simulink model "Appl_HeatAdj_CtrlModel"  (R2018b)
settings: configuration reference "CodeConfig_10_ms" (kept outside this file)
undefined symbols (not defined in the file): CAL_LEVEL3_TIMEOUT, CAL_SW_20min_TIMEOUT, D_1stLevel_36, D_2ndLevel_39, D_3rdLevel_45, D_3rdLevel_48, D_DRVHEAT_PID_D, D_DRVHEAT_PID_I, D_DRVHEAT_PID_P, D_HEAT_HEAT_DEF, D_SwsLevel_Temp, FALSE, TRUE
libraries: DareLib x111, simulink x1
(part 4 of 6)

== stateflow chart Appl_HeatAdj_CtrlModel/LogicCtrl/LocalAdjustCtrl/LimitDeal/LevelLimitFunction/LevelLimit ==
  state Default
    en:
    Level = enHeatLvlSts.EN_HEAT_LVL_OFF;
  state Run
    en:
    Level = OriginalLevel;
    CANStopReason = enHeatStopReason.EN_HEAT_STOP_R_NONE;
    du:
    Level = OriginalLevel;
  state ForbidStatus
    en:
    Level = enHeatLvlSts.EN_HEAT_LVL_OFF;
    CANStopReason = StopReason;
    //暂时屏蔽，查看是否需要一直保存禁能原因
    ex:
    StopReason = enHeatStopReason.EN_HEAT_STOP_R_NONE;
    (default) -> (junction 34)
    ForbidStatus -> (junction 34) [order 1]
    (junction 34) -> (junction 37) [order 1] : /*存在故障*/
        | [TRUE == Error]
    (junction 34) -> (junction 41) [order 2]
    (junction 37) -> (junction 39) : {StopReason = enHeatStopReason.EN_HEAT_STOP_R_FAULT;}
    (junction 39) -> (junction 41)
    (junction 41) -> (junction 44)
    (junction 44) -> (junction 46) [order 1] : /*互斥命令有效*/
        | [TRUE == OppositeCmd]
    (junction 44) -> (junction 50) [order 2]
    (junction 46) -> (junction 48) : {StopReason = enHeatStopReason.EN_HEAT_STOP_R_CMD;}
    (junction 48) -> (junction 50)
    (junction 50) -> (junction 62)
    (junction 62) -> (junction 60) [order 1] : /*恢复出厂*/
        | [TRUE == Heat_RecoverDefaultFlag]
    (junction 62) -> (junction 55) [order 2]
    (junction 60) -> (junction 58) : {StopReason = enHeatStopReason.EN_HEAT_STOP_R_FACTORY;}
    (junction 58) -> (junction 55)
    (junction 55) -> (junction 71)
    (junction 71) -> (junction 69) [order 1] : /*BM400掉线禁能*/
        | [TRUE == Heat_CanMessageLostFlag && enProjectType.EN_PROJECT_BM400 == CarType]
    (junction 71) -> (junction 67) [order 2]
    (junction 69) -> (junction 64) : {StopReason = enHeatStopReason.EN_HEAT_STOP_R_LOSS;}
    (junction 64) -> (junction 67)
    (junction 67) -> (junction 73)
  (default) -> Default
  ForbidStatus -> Default [order 1] : /*无用户请求，可准备下一轮禁能原因检测*/
      | [enHeatLvlSts.EN_HEAT_LVL_OFF == OriginalLevel]
  Default -> ForbidStatus : /*请求工作*/
      | [enHeatLvlSts.EN_HEAT_LVL_OFF != OriginalLevel]
  Run -> ForbidStatus [order 1] : /*存在故障*/
      | [TRUE == Error]
      | /StopReason = enHeatStopReason.EN_HEAT_STOP_R_FAULT;
  Run -> ForbidStatus [order 2] : /*互斥命令有效*/
      | [TRUE == OppositeCmd]
      | /StopReason = enHeatStopReason.EN_HEAT_STOP_R_CMD;
  Run -> ForbidStatus [order 3] : /*恢复出厂*/
      | [TRUE == Heat_RecoverDefaultFlag]
      | /StopReason = enHeatStopReason.EN_HEAT_STOP_R_FACTORY;
  Run -> ForbidStatus [order 4] : /*BM400掉线禁能*/
      | [TRUE == Heat_CanMessageLostFlag && enProjectType.EN_PROJECT_BM400 == CarType]
      | /StopReason = enHeatStopReason.EN_HEAT_STOP_R_LOSS;
  ForbidStatus -> Run [order 2] : /*无故障
      | && 互斥命令无效
      | && 无恢复出厂命令
      | && （BM400控制报文在线 || 非BM400车型）*/
      | [TRUE != Error ...
      | && TRUE != OppositeCmd ...
      | && TRUE != Heat_RecoverDefaultFlag ...
      | && ((FALSE == Heat_CanMessageLostFlag && enProjectType.EN_PROJECT_BM400 == CarType) ...
      | || (enProjectType.EN_PROJECT_BM400 != CarType))]
      | /StopReason = enHeatStopReason.EN_HEAT_STOP_R_NONE
  data: Level output Enum: enHeatLvlSts; StopReason output Enum: enHeatStopReason; OriginalLevel input Enum: enHeatLvlSts; Error input uint8; CarType input Enum: enProjectType; TRUE parameter; OppositeCmd input uint8; Heat_CanMessageLostFlag input uint8; Heat_RecoverDefaultFlag input uint8; FALSE parameter; CANStopReason output Enum: enHeatStopReason

== stateflow chart Appl_HeatAdj_CtrlModel/LogicCtrl/LocalAdjustCtrl/LimitDeal/TimeoutFunction1/Timeout ==
  state Ts = D_HAL_GET_CUR_MS_TS [function]
  state OutTs = TimeDiffTs(lastTs,Ts) [function]
  state TimeCountStatus
    state TimeoutSts
      en:
      Level = enHeatLvlSts.EN_HEAT_LVL_OFF;
      du:
      Level = enHeatLvlSts.EN_HEAT_LVL_OFF;
      ex:
      Timer = 0;
    state Init
      en:
      Level = InLevel;
      Timer = D_HAL_GET_CUR_MS_TS();
      du:
      Level = InLevel;
      ex:
      Timer = D_HAL_GET_CUR_MS_TS();
    (default) -> Init
    Init -> TimeoutSts [order 1] : [TimeDiffTs(Timer,D_HAL_GET_CUR_MS_TS()) >= MaxTime]
        | /TimeoutFlag = TRUE;
    TimeoutSts -> Init : [hasChangedFrom(InLevel,enHeatLvlSts.EN_HEAT_LVL_OFF)]
    Init -> Init [order 2] : [hasChangedFrom(InLevel,enHeatLvlSts.EN_HEAT_LVL_OFF)]
  state Default
    en:
    Level = InLevel;
    du:
    Level = InLevel;
  (default) -> Default
  Default -> TimeCountStatus : /*有超时配置
      | && 启动加热&&有时间值 */
      | [TRUE == TimeoutPrm ...
      | && enHeatLvlSts.EN_HEAT_LVL_OFF != InLevel ...
      | && 0 != MaxTime]
  TimeCountStatus -> Default : /*无超时配置*/
      | [TRUE != TimeoutPrm || 0 == MaxTime]
      | /TimeoutFlag = FALSE;
  data: Ts function_output; lastTs function_input; Ts function_input; OutTs function_output; TimeoutPrm input uint8; TimeoutFlag output uint8; FALSE parameter; TRUE parameter; InLevel input Enum: enHeatLvlSts; MaxTime input uint32; Timer local uint32; Level output Enum: enHeatLvlSts

== stateflow chart Appl_HeatAdj_CtrlModel/UpDataInputInfo/InputSignalProcess/RemoteMode/RemoteMode ==
  state Default
    en:
    RemoteModeFlag = FALSE;
  state ValidSts
    en:
    RemoteModeFlag = TRUE;
  (default) -> Default
  Default -> ValidSts : /*平台远程配置字使能
      | && 远程报文在线
      | && 车辆变为远程模式*/
      | [TRUE == HeatAdj_RemoteEnableConfig ...
      | && FALSE == HeatAdj_RemoteMsgLostFlag ...
      | && HeatAdj_TboxRemoteSts == TRUE ]
  ValidSts -> Default : /*平台远程配置字禁能
      | || 远程报文掉线
      | || （车辆变为非远程模式&&远程报文在线）*/
      | [FALSE == HeatAdj_RemoteEnableConfig ...
      | || TRUE == HeatAdj_RemoteMsgLostFlag ...
      | || (HeatAdj_TboxRemoteSts == FALSE ...
      | && FALSE == HeatAdj_RemoteMsgLostFlag)]
  data: FALSE parameter; TRUE parameter; RemoteModeFlag output uint8; HeatAdj_RemoteEnableConfig input; HeatAdj_TboxRemoteSts input; HeatAdj_RemoteMsgLostFlag input

== stateflow chart Appl_HeatAdj_CtrlModel/UpDataInputInfo/InputSignalProcess/EngineRunning/EngineStatus ==
  state Default
    en:
    EngineRunningFlag = FALSE;
  state ValidSts
    en:
    EngineRunningFlag = TRUE;
  (default) -> Default
  Default -> ValidSts : /*（平台发动机配置字使能
      | && P20车型配置字禁能
      | && 发动机状态为运行）
      | || 平台发动机配置字禁能
      | || 非P20车型*/
      | [(TRUE == HeatAdj_PlatformEngineEnableConfig ...
      | && FALSE == HeatAdj_P20_PHEV_EngineCfg ...
      | && enEngineType.EN_ENGINE_RUNNING == HeatAdj_ECMD_EngineStatus) ...
      | || FALSE == HeatAdj_PlatformEngineEnableConfig ...
      | || enProjectType.EN_PROJECT_P20 != HeatAdj_CarType]
  ValidSts -> Default : /*平台发动机配置字使能
      | && (P20车型配置字使能
      | || 发动机状态非运行)*/
      | [TRUE == HeatAdj_PlatformEngineEnableConfig ...
      | && (TRUE == HeatAdj_P20_PHEV_EngineCfg ...
      | || (enEngineType.EN_ENGINE_RUNNING != HeatAdj_ECMD_EngineStatus ...
      | && enEngineType.EN_ENGINE_RESERVED != HeatAdj_ECMD_EngineStatus))]
  data: FALSE parameter; TRUE parameter; EngineRunningFlag output uint8; HeatAdj_PlatformEngineEnableConfig input; HeatAdj_P20_PHEV_EngineCfg input; HeatAdj_ECMD_EngineStatus input; HeatAdj_CarType input

== stateflow chart Appl_HeatAdj_CtrlModel/UpDataInputInfo/InputSignalProcess/VentilateMessage/VentilateMessage ==
  state VenSts = OppositeMessageDeal(CarTypeCfg,RemoteModeFlag,HMI_Message,Tbox_Message,VentCfg) [function]
  state VenSts = OppositeMessageDeal1(CarTypeCfg,RemoteModeFlag,HMI_Message,Tbox_Message,VentCfg) [function]
  state VenSts = OppositeMessageDeal2(CarTypeCfg,RemoteModeFlag,HMI_Message,Tbox_Message,VentCfg) [function]
  state run
    du:
    DriverVentilateValid = OppositeMessageDeal(HeatAdj_CarType,RemoteModeFlag,HeatAdj_Driver_HMI_VentilateMsg,HeatAdj_Driver_Tbox_VentilateMsg,DrVentConfig);
    PassengerVentilateValid = OppositeMessageDeal1(HeatAdj_CarType,RemoteModeFlag,HeatAdj_Passenger_HMI_VentilateMsg,HeatAdj_Passenger_Tbox_VentilateMsg,PaVentConfig);
    ThirdVentilateValid = OppositeMessageDeal2(HeatAdj_CarType,RemoteModeFlag,HeatAdj_Third_HMI_VentilateMsg,HeatAdj_Third_Tbox_VentilateMsg,ThirdVentConfig);
  (default) -> run
  data: CarTypeCfg function_input; RemoteModeFlag function_input; HMI_Message function_input; Tbox_Message function_input; VenSts function_output; VentCfg function_input; CarTypeCfg function_input; RemoteModeFlag function_input; HMI_Message function_input; Tbox_Message function_input; VenSts function_output; VentCfg function_input; CarTypeCfg function_input; RemoteModeFlag function_input; HMI_Message function_input; Tbox_Message function_input; VenSts function_output; VentCfg function_input; DriverVentilateValid output uint8; PassengerVentilateValid output uint8; ThirdVentilateValid output uint8; HeatAdj_CarType input; HeatAdj_Driver_HMI_VentilateMsg input; HeatAdj_Driver_Tbox_VentilateMsg input; HeatAdj_Passenger_HMI_VentilateMsg input; HeatAdj_Passenger_Tbox_VentilateMsg input; HeatAdj_Third_HMI_VentilateMsg input; HeatAdj_Third_Tbox_VentilateMsg input; RemoteModeFlag input; DrVentConfig input; PaVentConfig input; ThirdVentConfig input

== stateflow chart Appl_HeatAdj_CtrlModel/UpDataInputInfo/InputSignalProcess/VentilateMessage/VentilateMessage/OppositeMessageDeal/OppositeMessageDeal ==
  state HMIMessageDeal [parallel]
    settings: executionOrder=1
    state HMIInit
      en:
      TempHMI = FALSE;
    state HMIValid
      en:
      TempHMI = TRUE;
    (default) -> HMIInit
    HMIInit -> HMIValid : /*HMI档位请求有效*/
        | [(enProjectType.EN_PROJECT_BM400 != CarTypeCfg && (0x1 == HMI_Message || 0x2 == HMI_Message || 0x3 == HMI_Message || 0x5 == HMI_Message)) ...
        | || (enProjectType.EN_PROJECT_BM400 == CarTypeCfg && (0x8 == HMI_Message || 0x9 == HMI_Message || 0xA == HMI_Message))]
    HMIValid -> HMIInit : /*HMI报文关闭*/
        | [(enProjectType.EN_PROJECT_BM400 != CarTypeCfg && 0x1 != HMI_Message && 0x2 != HMI_Message && 0x3 != HMI_Message && 0x5 != HMI_Message) ...
        | || (enProjectType.EN_PROJECT_BM400 == CarTypeCfg && 0x8 != HMI_Message && 0x9 != HMI_Message && 0xA != HMI_Message)]
  state TboxMessageDeal [parallel]
    settings: executionOrder=2
    state TboxValid
      en:
      TempTbox = TRUE;
    state TboxInit
      en:
      TempTbox = FALSE;
    (default) -> TboxInit
    TboxInit -> TboxValid : /*Tbox档位请求有效*/
        | [(TRUE == RemoteModeFlag) ...
        | && (0x1 == Tbox_Message || 0x2 == Tbox_Message || 0x3 == Tbox_Message)]
    TboxValid -> TboxInit : /*Tbox报文关闭*/
        | [FALSE == RemoteModeFlag ...
        | || (0x1 != Tbox_Message && 0x2 != Tbox_Message && 0x3 != Tbox_Message)]
  state VenStatus [parallel]
    settings: executionOrder=3
    state TotalValid
      en:
      VenSts = TRUE;
    state TotalInit
      en:
      VenSts = FALSE;
    (default) -> TotalInit
    TotalInit -> TotalValid : /*档位请求有效 且配置有效*/
        | [(TRUE == TempHMI || TRUE == TempTbox) && VentCfg == TRUE]
    TotalValid -> TotalInit : /* 档位请求无效 或配置无效 */
        | [(FALSE == TempHMI && FALSE == TempTbox) || VentCfg == FALSE]
  data: CarTypeCfg input Enum: enProjectType; RemoteModeFlag input uint8; HMI_Message input uint8; Tbox_Message input uint8; VenSts output uint8; TempHMI local uint8; TRUE parameter; FALSE parameter; TempTbox local uint8; VentCfg input uint8

== stateflow chart Appl_HeatAdj_CtrlModel/UpDataInputInfo/InputSignalProcess/EorrorProcess/EorrorProcess ==
  state HeatError = ErrorFunction2(FirstFaultSts,SecondFaultSts) [function]
  state HeatError = ErrorFunction3(FirstFaultSts,SecondFaultSts) [function]
  state HeatError = ErrorFunction1(FirstFaultSts,SecondFaultSts) [function]
  state HeatError = ErrorFunction4(FirstFaultSts,SecondFaultSts) [function]
  state HeatError = ErrorFunction(FirstFaultSts,SecondFaultSts) [function]
  state HeatError = ErrorFunction5(FirstFaultSts,SecondFaultSts) [function]
  state run
    du:
    DriverHeatError = ErrorFunction(HeatAdj_DriverCmdFaultSts,HeatAdj_DriverNTCFaultSts);
    PassengerHeatError = ErrorFunction1(HeatAdj_PassengerCmdFaultSts,HeatAdj_PassengerNTCFaultSts);
    ThirdHeatError = ErrorFunction2(HeatAdj_ThirdCmdFaultSts,HeatAdj_ThirdNTCFaultSts);
    DriverHeatErrorDtc = ErrorFunction3(HeatAdj_DriverCmdFaultSts4DTC,HeatAdj_DriverNTCFaultSts);
    PassengerHeatErrorDtc = ErrorFunction4(HeatAdj_PassengerCmdFaultSts4DTC,HeatAdj_PassengerNTCFaultSts);
    ThirdHeatErrorDtc = ErrorFunction5(HeatAdj_ThirdCmdFaultSts4DTC,HeatAdj_ThirdNTCFaultSts);
  (default) -> run
  data: FirstFaultSts function_input; SecondFaultSts function_input; HeatError function_output; FirstFaultSts function_input; SecondFaultSts function_input; HeatError function_output; FirstFaultSts function_input; SecondFaultSts function_input; HeatError function_output; FirstFaultSts function_input; SecondFaultSts function_input; HeatError function_output; FirstFaultSts function_input; SecondFaultSts function_input; HeatError function_output; FirstFaultSts function_input; SecondFaultSts function_input; HeatError function_output; DriverHeatError output uint8; PassengerHeatError output uint8; ThirdHeatError output uint8; HeatAdj_DriverCmdFaultSts input; HeatAdj_DriverNTCFaultSts input; HeatAdj_PassengerCmdFaultSts input; HeatAdj_PassengerNTCFaultSts input; HeatAdj_ThirdCmdFaultSts input; HeatAdj_ThirdNTCFaultSts input; DriverHeatErrorDtc output uint8; PassengerHeatErrorDtc output uint8; ThirdHeatErrorDtc output uint8; HeatAdj_DriverCmdFaultSts4DTC input; HeatAdj_PassengerCmdFaultSts4DTC input; HeatAdj_ThirdCmdFaultSts4DTC input

== stateflow chart Appl_HeatAdj_CtrlModel/UpDataInputInfo/InputSignalProcess/EorrorProcess/EorrorProcess/ErrorFunction/OppositeMessageDeal ==
  state Default
    en:
    HeatErr = FALSE;
  state Fault
    en:
    HeatErr = TRUE;
  (default) -> Default
  Default -> Fault : /*任一故障输入*/
      | [FALSE != FirstFaultSts ...
      | || FALSE != SecondFaultSts]
  Fault -> Default : /*无故障输入*/
      | [FALSE == FirstFaultSts ...
      | && FALSE == SecondFaultSts]
  data: TRUE parameter; FALSE parameter; FirstFaultSts input uint8; SecondFaultSts input uint8; HeatErr output uint8

== stateflow chart Appl_HeatAdj_CtrlModel/LogicCtrl/LocalAdjustCtrl/LimitDeal/StopFunction/StopFunction ==
  state ValidSts
    en,du:
    StopReason = enHeatStopReason.EN_HEAT_STOP_R_TIME;
    CANStopReason = enHeatStopReason.EN_HEAT_STOP_R_TIME;
  state Default
    en,du:
    StopReason = ComStop;
    CANStopReason = ComCANStop;
  (default) -> Default
  Default -> ValidSts : /*无通用限制
      | &&超时限制有效*/
      | [enHeatStopReason.EN_HEAT_STOP_R_NONE == ComStop ...
      | && TRUE  == Timeout]
  ValidSts -> Default : /*无超时限制*/
      | [FALSE  == Timeout]
  data: FALSE parameter; StopReason output Enum: enHeatStopReason; ComStop input Enum: enHeatStopReason; Timeout input uint8; TRUE parameter; ComCANStop input; CANStopReason output Enum: enHeatStopReason

== stateflow chart Appl_HeatAdj_CtrlModel/LogicCtrl/LocalAdjustCtrl/LimitDeal/DiagnoseFunction/Diagnose ==
  state Diagnose
    (default) -> (junction 6)
    Diagnose -> (junction 6)
    (junction 6) -> (junction 8) [order 1] : /* 无诊断指令 */
        | [0 == DiagCommand || DiagCommand > (enHeatLvlSts.EN_HEAT_LVL_3 + 1)]
    (junction 6) -> (junction 14) [order 2] : {Level = DiagCommand - 1;
        | Type = enHeatType.EN_HEAT_TYPE_DIAG;}
    (junction 8) -> (junction 10) : {Level = InLevel;
        | Type = CurrentType;}
    (junction 10) -> (junction 14)
    (junction 14) -> (junction 17)
  (default) -> Diagnose
  data: DiagCommand input uint8; InLevel input Enum: enHeatLvlSts; CurrentType input Enum: enHeatType; Level output Enum: enHeatLvlSts; Type output Enum: enHeatType

== stateflow chart Appl_HeatAdj_CtrlModel/LogicCtrl/LocalAdjustCtrl/OutputDeal ==
  state CANOutputDeal [parallel]
    settings: executionOrder=1
    state ProjectP20
      en:
      /*Initial Value(Hex)初始值:0x0*/
      OutDrCANHeatLevel = 0;
      OutPaCANHeatLevel =  0;
      Out3rdCANHeatLevel = 0;
      state Drv [parallel]
        settings: executionOrder=1
        state Run
          en,du:
          /*0x0:Level 1  1档
          0x1:Level 2   2档
          0x2:Level 3   3档*/
          OutDrCANHeatLevel = DiagDrHeatLevel - 1;
          LocalDrRunState = TRUE;
        state Init
          en:
          LocalDrRunState = FALSE;
        (default) -> CANOutputDeal.ProjectP20.Drv.Init
        CANOutputDeal.ProjectP20.Drv.Run -> CANOutputDeal.ProjectP20.Drv.Init : /* 主驾加热无指令 ,档位反馈关闭前档位*/
            | [enHeatLvlSts.EN_HEAT_LVL_OFF == DiagDrHeatLevel]
        CANOutputDeal.ProjectP20.Drv.Init -> CANOutputDeal.ProjectP20.Drv.Run : /* 主驾加热指令 */
            | [enHeatLvlSts.EN_HEAT_LVL_OFF != DiagDrHeatLevel]
      state Pas [parallel]
        settings: executionOrder=2
        state Run
          en,du:
          /*0x0:Level 1  1档
          0x1:Level 2   2档
          0x2:Level 3   3档*/
          OutPaCANHeatLevel = DiagPaHeatLevel - 1;
          LocalPaRunState = TRUE;
        state Init
          en:
          LocalPaRunState = FALSE;
        (default) -> CANOutputDeal.ProjectP20.Pas.Init
        CANOutputDeal.ProjectP20.Pas.Run -> CANOutputDeal.ProjectP20.Pas.Init : /* 副驾加热无指令 ,档位反馈关闭前档位*/
            | [enHeatLvlSts.EN_HEAT_LVL_OFF == DiagPaHeatLevel]
        CANOutputDeal.ProjectP20.Pas.Init -> CANOutputDeal.ProjectP20.Pas.Run : /* 副驾加热指令 */
            | [enHeatLvlSts.EN_HEAT_LVL_OFF != DiagPaHeatLevel]
      state Treble [parallel]
        settings: executionOrder=3
        state Run
          en,du:
          /*0x0:Level 1  1档
          0x1:Level 2   2档
          0x2:Level 3   3档*/
          Out3rdCANHeatLevel = Diag3rdHeatLevel - 1;
          Local3rdRunState = TRUE;
        state Init
          en:
          Local3rdRunState = FALSE;
        (default) -> CANOutputDeal.ProjectP20.Treble.Init
        CANOutputDeal.ProjectP20.Treble.Run -> CANOutputDeal.ProjectP20.Treble.Init : /* 三排加热无指令 ,档位反馈关闭前档位*/
            | [enHeatLvlSts.EN_HEAT_LVL_OFF == Diag3rdHeatLevel]
        CANOutputDeal.ProjectP20.Treble.Init -> CANOutputDeal.ProjectP20.Treble.Run : /* 三排加热无指令 */
            | [enHeatLvlSts.EN_HEAT_LVL_OFF != Diag3rdHeatLevel]
    state Default
      en:
      OutDrCANHeatLevel = DiagDrHeatLevel;
      OutPaCANHeatLevel = DiagPaHeatLevel;
      Out3rdCANHeatLevel = Diag3rdHeatLevel;
      OutDrRunState = FALSE;
      OutPaRunState = FALSE;
      Out3rdRunState = FALSE;
      LocalDrRunState = FALSE;
      LocalPaRunState = FALSE;
      Local3rdRunState = FALSE;
      du:
      OutDrCANHeatLevel = DiagDrHeatLevel;
      OutPaCANHeatLevel = DiagPaHeatLevel;
      Out3rdCANHeatLevel = Diag3rdHeatLevel;
      OutDrRunState = FALSE;
      OutPaRunState = FALSE;
      Out3rdRunState = FALSE;
      LocalDrRunState = FALSE;
      LocalPaRunState = FALSE;
      Local3rdRunState = FALSE;
    (default) -> Default
    Default -> ProjectP20 : /* P20的车型 */
        | [enProjectType.EN_PROJECT_P20 == CarTypeCfg]
    ProjectP20 -> Default : /* 非P20车型 */
        | [enProjectType.EN_PROJECT_P20 != CarTypeCfg]
  state AcquireTemp [parallel]
    en:
    DrAimTemp = TempFunction(DiagDrHeatLevel,HeatAdj_CarType,FALSE);
    PaAimTemp = TempFunction1(DiagPaHeatLevel,HeatAdj_CarType,FALSE);
    ThirdAimTemp = TempFunction2(Diag3rdHeatLevel,HeatAdj_CarType,TRUE);
    du:
    DrAimTemp = TempFunction(DiagDrHeatLevel,HeatAdj_CarType,FALSE);
    PaAimTemp = TempFunction1(DiagPaHeatLevel,HeatAdj_CarType,FALSE);
    ThirdAimTemp = TempFunction2(Diag3rdHeatLevel,HeatAdj_CarType,TRUE);
    settings: executionOrder=5
  state TempHardwareOutput [parallel]
    en:
    [HeatAdj_DRHeatIo,HeatAdj_DRHeatPwmCnt] = HeatOutFunction(DrAimTemp,HeatAdj_DrHeatNtcAdc,DiagDrHeatLevel);
    [HeatAdj_PAHeatIo,HeatAdj_PAHeatPwmCnt] = HeatOutFunction1(PaAimTemp,HeatAdj_PaHeatNtcAdc,DiagPaHeatLevel);
    [HeatAdj_ThirdHeatIo,HeatAdj_ThirdHeatPwmCnt,SwTimeout,Sw20minTimerOut] = HeatOutFunction2(ThirdAimTemp,HeatAdj_ThirdHeatNtcAdc,Diag3rdHeatLevel,SwHeatRunMaxTime);
    du:
    [HeatAdj_DRHeatIo,HeatAdj_DRHeatPwmCnt] = HeatOutFunction(DrAimTemp,HeatAdj_DrHeatNtcAdc,DiagDrHeatLevel);
    [HeatAdj_PAHeatIo,HeatAdj_PAHeatPwmCnt] = HeatOutFunction1(PaAimTemp,HeatAdj_PaHeatNtcAdc,DiagPaHeatLevel);
    [HeatAdj_ThirdHeatIo,HeatAdj_ThirdHeatPwmCnt,SwTimeout,Sw20minTimerOut] = HeatOutFunction2(ThirdAimTemp,HeatAdj_ThirdHeatNtcAdc,Diag3rdHeatLevel,SwHeatRunMaxTime);
    settings: executionOrder=6
  state AimTemp = TempFunction(AimLevel,ProjectType,ThirdHeat) [function]
  state AimTemp = TempFunction1(AimLevel,ProjectType,ThirdHeat) [function]
  state AimTemp = TempFunction2(AimLevel,ProjectType,ThirdHeat) [function]
  state DrErr [parallel]
    settings: executionOrder=2
    state FalseSts
      en:
      OutDrRunState = LocalDrRunState;
      du:
      OutDrRunState = LocalDrRunState;
    state ErrSts
      en:
      OutDrRunState = 2;
      du:
      OutDrRunState = 2;
    (default) -> DrErr.FalseSts
    DrErr.FalseSts -> DrErr.ErrSts : /* 无指令 且存在故障 */
        | [LocalDrRunState == FALSE ...
        | &&DriverHeatErrorDtc == TRUE]
    DrErr.ErrSts -> DrErr.FalseSts : /*无故障 或RUN状态 */
        | [LocalDrRunState == TRUE ...
        | || DriverHeatErrorDtc == FALSE]
  state PaErr [parallel]
    settings: executionOrder=3
    state FalseSts
      en:
      OutPaRunState = LocalPaRunState;
      du:
      OutPaRunState = LocalPaRunState;
    state ErrSts
      en:
      OutPaRunState = 2;
      du:
      OutPaRunState = 2;
    (default) -> PaErr.FalseSts
    PaErr.FalseSts -> PaErr.ErrSts : /* 无指令 且存在故障 */
        | [LocalPaRunState == FALSE ...
        | && PassengerHeatErrorDtc == TRUE]
    PaErr.ErrSts -> PaErr.FalseSts : /*无故障 或RUN状态 */
        | [LocalPaRunState == TRUE ...
        | || PassengerHeatErrorDtc == FALSE]
  state [HeatOutGpio,HeatOutPwmCnt] = HeatOutFunction(SetTemp,CurrentTemp,HeatLvl) [function]
  state [HeatOutGpio,HeatOutPwmCnt] = HeatOutFunction1(SetTemp,CurrentTemp,HeatLvl) [function]
  state [HeatOutGpio,HeatOutPwmCnt,SwTimeoutFlag,Sw20minTimer] = HeatOutFunction2(SetTemp,CurrentTemp,HeatLvl,MaxTime) [function]
  state ThirdErr [parallel]
    settings: executionOrder=4
    state FalseSts
      en:
      Out3rdRunState = Local3rdRunState;
      du:
      Out3rdRunState = Local3rdRunState;
    state ErrSts
      en:
      Out3rdRunState = 2;
      du:
      Out3rdRunState = 2;
    (default) -> ThirdErr.FalseSts
    ThirdErr.FalseSts -> ThirdErr.ErrSts : /* 无指令 且存在故障 */
        | [Local3rdRunState == FALSE ...
        | && ThirdHeatErrorDtc == TRUE]
    ThirdErr.ErrSts -> ThirdErr.FalseSts : /*无故障 或RUN状态 */
        | [Local3rdRunState == TRUE ...
        | || ThirdHeatErrorDtc == FALSE]
  data: AimLevel function_input; AimTemp function_output; ProjectType function_input; ThirdHeat function_input; AimLevel function_input; AimTemp function_output; ProjectType function_input; ThirdHeat function_input; AimLevel function_input; AimTemp function_output; ProjectType function_input; ThirdHeat function_input; SetTemp function_input; CurrentTemp function_input; HeatOutGpio function_output; HeatLvl function_input; HeatOutPwmCnt function_output; SetTemp function_input; CurrentTemp function_input; HeatOutGpio function_output; HeatLvl function_input; HeatOutPwmCnt function_output; SetTemp function_input; CurrentTemp function_input; HeatOutGpio function_output; HeatLvl function_input; HeatOutPwmCnt function_output; SwTimeoutFlag function_output; Sw20minTimer function_output; MaxTime function_input uint32; OutDrCANHeatLevel output Enum: enHeatLvlSts; OutPaCANHeatLevel output Enum: enHeatLvlSts; Out3rdCANHeatLevel output Enum: enHeatLvlSts; CarTypeCfg input; DiagDrHeatLevel input; DiagPaHeatLevel input; Diag3rdHeatLevel input; DrAimTemp local uint16; PaAimTemp local uint16; ThirdAimTemp local uint16; HeatAdj_DrHeatNtcAdc input; HeatAdj_PaHeatNtcAdc input; HeatAdj_ThirdHeatNtcAdc input; HeatAdj_DRHeatIo output Enum: enHeatIoSts; HeatAdj_PAHeatIo output Enum: enHeatIoSts; HeatAdj_ThirdHeatIo output Enum: enHeatIoSts; HeatAdj_DRHeatPwmCnt output uint8; HeatAdj_PAHeatPwmCnt output uint8; HeatAdj_ThirdHeatPwmCnt output uint8; FALSE parameter; OutDrRunState output uint8; OutPaRunState output uint8; Out3rdRunState output uint8; TRUE parameter; LocalDrRunState local uint8; LocalPaRunState local uint8; Local3rdRunState local uint8; DriverHeatErrorDtc input; PassengerHeatErrorDtc input; ThirdHeatErrorDtc input; HeatAdj_CarType input; SwTimeout output uint8; SwHeatRunMaxTime input; Sw20minTimerOut output uint32

== stateflow chart Appl_HeatAdj_CtrlModel/LogicCtrl/LocalAdjustCtrl/OutputDeal/TempFunction/TempFunction ==
  state Ts = D_HAL_GET_CUR_MS_TS [function]
  state OutTs = TimeDiffTs(lastTs,Ts) [function]
  state TempLvl
    (default) -> (junction 39)
    TempLvl -> (junction 39)
    (junction 39) -> (junction 41) [order 1] : /* P20方向盘加热等级 */
        | [enProjectType.EN_PROJECT_P20 == ProjectType ...
        | && TRUE == ThirdHeat]
    (junction 39) -> (junction 6) [order 2]
    (junction 41) -> (junction 43) : {AimTemp = D_SwsLevel_Temp;
        | TimeCnt = D_HAL_GET_CUR_MS_TS();}
    (junction 6) -> (junction 8) [order 1] : /* 等级1 */
        | [enHeatLvlSts.EN_HEAT_LVL_1 == AimLevel]
    (junction 6) -> (junction 10) [order 2]
    (junction 8) -> (junction 24) : {AimTemp = D_1stLevel_36;
        | TimeCnt = D_HAL_GET_CUR_MS_TS();}
    (junction 10) -> (junction 12) [order 1] : /* 等级2 */
        | [enHeatLvlSts.EN_HEAT_LVL_2 == AimLevel]
    (junction 10) -> (junction 14) [order 2]
    (junction 12) -> (junction 22) : {AimTemp = D_2ndLevel_39;
        | TimeCnt = D_HAL_GET_CUR_MS_TS();}
    (junction 14) -> (junction 16) [order 1] : /* 等级3 */
        | [enHeatLvlSts.EN_HEAT_LVL_3 == AimLevel]
    (junction 14) -> (junction 18) [order 2] : {AimTemp = 0;
        | TimeCnt = D_HAL_GET_CUR_MS_TS();}
    (junction 16) -> (junction 49)
    (junction 49) -> (junction 50) [order 1] : /* 小于13min 且为P20 且本次未降至 45度(防止32bit计数超时重新小于13min) */
        | [enProjectType.EN_PROJECT_P20 == ProjectType ...
        | && TimeDiffTs(TimeCnt,D_HAL_GET_CUR_MS_TS()) <= CAL_LEVEL3_TIMEOUT ...
        | && AimTemp != D_3rdLevel_45]
    (junction 49) -> (junction 20) [order 2] : {AimTemp = D_3rdLevel_45;}
    (junction 50) -> (junction 52) : {AimTemp = D_3rdLevel_48;}
    (junction 20) -> (junction 18)
    (junction 52) -> (junction 20)
    (junction 22) -> (junction 52)
    (junction 24) -> (junction 22)
    (junction 43) -> (junction 24)
    (junction 18) -> (junction 29)
  (default) -> TempLvl
  data: Ts function_output; lastTs function_input; Ts function_input; OutTs function_output; AimTemp output uint16; D_1stLevel_36 parameter; D_2ndLevel_39 parameter; AimLevel input Enum: enHeatLvlSts; ProjectType input uint8; ThirdHeat input uint8; D_SwsLevel_Temp parameter; TRUE parameter; TimeCnt local uint32; CAL_LEVEL3_TIMEOUT parameter; D_3rdLevel_45 parameter; D_3rdLevel_48 parameter

== stateflow chart Appl_HeatAdj_CtrlModel/LogicCtrl/LocalAdjustCtrl/OutputDeal/HeatOutFunction/HeatOut ==
  state PwmCnt = PidGetPwm(CurrentTemp,SetTemp) [function]
  state Controll
    state None
      en:
      du:
      HeatOutGpio = OFF;
      HeatOutPwmCnt = 0;
      TimeCnt = 0;
    state AllOut
      en:
      du:
      HeatOutGpio = ON;
      HeatOutPwmCnt =100;
      TimeCnt = 0;
    state PwmOut
      en:
      HeatOutPwmCnt = PidGetPwm(CurrentTemp,SetTemp);
      (default) -> (junction 11)
      PwmOut -> (junction 11) [order 1]
      (junction 11) -> (junction 12) [order 1] : /* 100计数 */
          | [TimeCnt <= 100]
      (junction 11) -> (junction 15) [order 2] : /* 计算pid 算pwm */
          | {TimeCnt = 0;
          | HeatOutPwmCnt = PidGetPwm(CurrentTemp,SetTemp);}
      (junction 12) -> (junction 13) : {TimeCnt += 1;}
      (junction 13) -> (junction 14) [order 1] : [TimeCnt <= HeatOutPwmCnt]
      (junction 13) -> (junction 16) [order 2] : /* 引脚拉低 */
          | {HeatOutGpio = OFF;}
      (junction 14) -> (junction 17) : /* 引脚拉高 */
          | {HeatOutGpio = ON;}
      (junction 16) -> (junction 15)
      (junction 17) -> (junction 16)
      (junction 15) -> (junction 18)
    (default) -> None
    None -> AllOut [order 1] : /* 加热误差在3度 全开 */
        | [enHeatLvlSts.EN_HEAT_LVL_OFF < HeatLvl ...
        | && SetTemp > CurrentTemp ...
        | && (SetTemp - CurrentTemp) >= D_HEAT_HEAT_DEF]
    AllOut -> None [order 1] : /*全开 进 关 */
        | [SetTemp <= CurrentTemp ...
        | || enHeatLvlSts.EN_HEAT_LVL_OFF == HeatLvl]
    PwmOut -> None [order 1] : /* PID 进 关 */
        | [SetTemp <= CurrentTemp ...
        | || enHeatLvlSts.EN_HEAT_LVL_OFF == HeatLvl]
    None -> PwmOut [order 2] : /* 关 进 PID */
        | [enHeatLvlSts.EN_HEAT_LVL_OFF < HeatLvl ...
        | && SetTemp > CurrentTemp ...
        | && (SetTemp - CurrentTemp) < D_HEAT_HEAT_DEF]
    PwmOut -> AllOut [order 2] : /* 加热误差在3度 全开 */
        | [enHeatLvlSts.EN_HEAT_LVL_OFF < HeatLvl ...
        | && SetTemp > CurrentTemp ...
        | && (SetTemp - CurrentTemp) >= D_HEAT_HEAT_DEF]
    AllOut -> PwmOut [order 2] : /* 全开 进PID */
        | [enHeatLvlSts.EN_HEAT_LVL_OFF < HeatLvl ...
        | && SetTemp > CurrentTemp ...
        | && (SetTemp - CurrentTemp) < D_HEAT_HEAT_DEF]
  data: CurrentTemp function_input; PwmCnt function_output; SetTemp function_input; CurrentTemp input uint16; HeatLvl input Enum: enHeatLvlSts; SetTemp input uint16; HeatOutGpio output uint8; TimeCnt local uint8; OFF parameter; ON parameter; D_HEAT_HEAT_DEF parameter; HeatOutPwmCnt output uint8

== stateflow chart Appl_HeatAdj_CtrlModel/UpDataInputInfo/InputSignalProcess/VentilateMessage/VentilateMessage/OppositeMessageDeal1/OppositeMessageDeal ==
  state HMIMessageDeal [parallel]
    settings: executionOrder=1
    state HMIInit
      en:
      TempHMI = FALSE;
    state HMIValid
      en:
      TempHMI = TRUE;
    (default) -> HMIInit
    HMIInit -> HMIValid : /*HMI档位请求有效*/
        | [(enProjectType.EN_PROJECT_BM400 != CarTypeCfg && (0x1 == HMI_Message || 0x2 == HMI_Message || 0x3 == HMI_Message || 0x5 == HMI_Message)) ...
        | || (enProjectType.EN_PROJECT_BM400 == CarTypeCfg && (0x8 == HMI_Message || 0x9 == HMI_Message || 0xA == HMI_Message))]
    HMIValid -> HMIInit : /*HMI报文关闭*/
        | [(enProjectType.EN_PROJECT_BM400 != CarTypeCfg && 0x1 != HMI_Message && 0x2 != HMI_Message && 0x3 != HMI_Message && 0x5 != HMI_Message) ...
        | || (enProjectType.EN_PROJECT_BM400 == CarTypeCfg && 0x8 != HMI_Message && 0x9 != HMI_Message && 0xA != HMI_Message)]
  state TboxMessageDeal [parallel]
    settings: executionOrder=2
    state TboxValid
      en:
      TempTbox = TRUE;
    state TboxInit
      en:
      TempTbox = FALSE;
    (default) -> TboxInit
    TboxInit -> TboxValid : /*Tbox档位请求有效*/
        | [(TRUE == RemoteModeFlag) ...
        | && (0x1 == Tbox_Message || 0x2 == Tbox_Message || 0x3 == Tbox_Message)]
    TboxValid -> TboxInit : /*Tbox报文关闭*/
        | [FALSE == RemoteModeFlag ...
        | || (0x1 != Tbox_Message && 0x2 != Tbox_Message && 0x3 != Tbox_Message)]
  state VenStatus [parallel]
    settings: executionOrder=3
    state TotalValid
      en:
      VenSts = TRUE;
    state TotalInit
      en:
      VenSts = FALSE;
    (default) -> TotalInit
    TotalInit -> TotalValid : /*档位请求有效 且配置有效*/
        | [(TRUE == TempHMI || TRUE == TempTbox) && VentCfg == TRUE]
    TotalValid -> TotalInit : /* 档位请求无效 或配置无效 */
        | [(FALSE == TempHMI && FALSE == TempTbox) || VentCfg == FALSE]
  data: CarTypeCfg input Enum: enProjectType; RemoteModeFlag input uint8; HMI_Message input uint8; Tbox_Message input uint8; VenSts output uint8; TempHMI local uint8; TRUE parameter; FALSE parameter; TempTbox local uint8; VentCfg input uint8

== stateflow chart Appl_HeatAdj_CtrlModel/LogicCtrl/LocalAdjustCtrl/OutputDeal/HeatOutFunction/HeatOut/PidGetPwm/Pid  ==
  (default) -> (junction 14)
  (junction 14) -> (junction 16) : /* 局部初始化 */
      | {Error = 0;
      | dError = 0;}
  (junction 16) -> (junction 20) : /* PID 计算 */
      | {Error = SetTemp - CurrentTemp;
      | SumError += Error;
      | dError = Error - LastError;
      | LastError = Error;
      | PwmCnt = (D_DRVHEAT_PID_P * Error)  + (D_DRVHEAT_PID_I *SumError) + (D_DRVHEAT_PID_D *  dError);}
  (junction 20) -> (junction 29) [order 1] : [PwmCnt > 100]
  (junction 20) -> (junction 27) [order 2]
  (junction 29) -> (junction 31) : {PwmCnt = 100;}
  (junction 31) -> (junction 27)
  (junction 27) -> (junction 34)
  data: dError local uint32; Error local uint32; CurrentTemp input uint16; SetTemp input uint16; PwmCnt output uint16; SumError local uint32; LastError local uint32; D_DRVHEAT_PID_P parameter; D_DRVHEAT_PID_I parameter; D_DRVHEAT_PID_D parameter

== stateflow chart Appl_HeatAdj_CtrlModel/UpDataInputInfo/InputSignalProcess/VentilateMessage/VentilateMessage/OppositeMessageDeal2/OppositeMessageDeal ==
  state HMIMessageDeal [parallel]
    settings: executionOrder=1
    state HMIInit
      en:
      TempHMI = FALSE;
    state HMIValid
      en:
      TempHMI = TRUE;
    (default) -> HMIInit
    HMIInit -> HMIValid : /*HMI档位请求有效*/
        | [(enProjectType.EN_PROJECT_BM400 != CarTypeCfg && (0x1 == HMI_Message || 0x2 == HMI_Message || 0x3 == HMI_Message || 0x5 == HMI_Message)) ...
        | || (enProjectType.EN_PROJECT_BM400 == CarTypeCfg && (0x8 == HMI_Message || 0x9 == HMI_Message || 0xA == HMI_Message))]
    HMIValid -> HMIInit : /*HMI报文关闭*/
        | [(enProjectType.EN_PROJECT_BM400 != CarTypeCfg && 0x1 != HMI_Message && 0x2 != HMI_Message && 0x3 != HMI_Message && 0x5 != HMI_Message) ...
        | || (enProjectType.EN_PROJECT_BM400 == CarTypeCfg && 0x8 != HMI_Message && 0x9 != HMI_Message && 0xA != HMI_Message)]
  state TboxMessageDeal [parallel]
    settings: executionOrder=2
    state TboxValid
      en:
      TempTbox = TRUE;
    state TboxInit
      en:
      TempTbox = FALSE;
    (default) -> TboxInit
    TboxInit -> TboxValid : /*Tbox档位请求有效*/
        | [(TRUE == RemoteModeFlag) ...
        | && (0x1 == Tbox_Message || 0x2 == Tbox_Message || 0x3 == Tbox_Message)]
    TboxValid -> TboxInit : /*Tbox报文关闭*/
        | [FALSE == RemoteModeFlag ...
        | || (0x1 != Tbox_Message && 0x2 != Tbox_Message && 0x3 != Tbox_Message)]
  state VenStatus [parallel]
    settings: executionOrder=3
    state TotalValid
      en:
      VenSts = TRUE;
    state TotalInit
      en:
      VenSts = FALSE;
    (default) -> TotalInit
    TotalInit -> TotalValid : /*档位请求有效 且配置有效*/
        | [(TRUE == TempHMI || TRUE == TempTbox) && VentCfg == TRUE]
    TotalValid -> TotalInit : /* 档位请求无效 或配置无效 */
        | [(FALSE == TempHMI && FALSE == TempTbox) || VentCfg == FALSE]
  data: CarTypeCfg input Enum: enProjectType; RemoteModeFlag input uint8; HMI_Message input uint8; Tbox_Message input uint8; VenSts output uint8; TempHMI local uint8; TRUE parameter; FALSE parameter; TempTbox local uint8; VentCfg input uint8

== stateflow chart Appl_HeatAdj_CtrlModel/UpDataInputInfo/InputSignalProcess/EorrorProcess/EorrorProcess/ErrorFunction1/OppositeMessageDeal ==
  state Default
    en:
    HeatErr = FALSE;
  state Fault
    en:
    HeatErr = TRUE;
  (default) -> Default
  Default -> Fault : /*任一故障输入*/
      | [FALSE != FirstFaultSts ...
      | || FALSE != SecondFaultSts]
  Fault -> Default : /*无故障输入*/
      | [FALSE == FirstFaultSts ...
      | && FALSE == SecondFaultSts]
  data: TRUE parameter; FALSE parameter; FirstFaultSts input uint8; SecondFaultSts input uint8; HeatErr output uint8

== stateflow chart Appl_HeatAdj_CtrlModel/UpDataInputInfo/InputSignalProcess/EorrorProcess/EorrorProcess/ErrorFunction2/OppositeMessageDeal ==
  state Default
    en:
    HeatErr = FALSE;
  state Fault
    en:
    HeatErr = TRUE;
  (default) -> Default
  Default -> Fault : /*任一故障输入*/
      | [FALSE != FirstFaultSts ...
      | || FALSE != SecondFaultSts]
  Fault -> Default : /*无故障输入*/
      | [FALSE == FirstFaultSts ...
      | && FALSE == SecondFaultSts]
  data: TRUE parameter; FALSE parameter; FirstFaultSts input uint8; SecondFaultSts input uint8; HeatErr output uint8

== stateflow chart Appl_HeatAdj_CtrlModel/LogicCtrl/LocalAdjustCtrl/LimitDeal/StopFunction1/StopFunction ==
  state ValidSts
    en,du:
    StopReason = enHeatStopReason.EN_HEAT_STOP_R_TIME;
    CANStopReason = enHeatStopReason.EN_HEAT_STOP_R_TIME;
  state Default
    en,du:
    StopReason = ComStop;
    CANStopReason = ComCANStop;
  (default) -> Default
  Default -> ValidSts : /*无通用限制
      | &&超时限制有效*/
      | [enHeatStopReason.EN_HEAT_STOP_R_NONE == ComStop ...
      | && TRUE  == Timeout]
  ValidSts -> Default : /*无超时限制*/
      | [FALSE  == Timeout]
  data: FALSE parameter; StopReason output Enum: enHeatStopReason; ComStop input Enum: enHeatStopReason; Timeout input uint8; TRUE parameter; ComCANStop input; CANStopReason output Enum: enHeatStopReason

== stateflow chart Appl_HeatAdj_CtrlModel/LogicCtrl/LocalAdjustCtrl/LimitDeal/StopFunction2/StopFunction ==
  state ValidSts
    en,du:
    StopReason = enHeatStopReason.EN_HEAT_STOP_R_TIME;
    CANStopReason = enHeatStopReason.EN_HEAT_STOP_R_TIME;
  state Default
    en,du:
    StopReason = ComStop;
    CANStopReason = ComCANStop;
  (default) -> Default
  Default -> ValidSts : /*无通用限制
      | &&超时限制有效*/
      | [enHeatStopReason.EN_HEAT_STOP_R_NONE == ComStop ...
      | && TRUE  == Timeout]
  ValidSts -> Default : /*无超时限制*/
      | [FALSE  == Timeout]
  data: FALSE parameter; StopReason output Enum: enHeatStopReason; ComStop input Enum: enHeatStopReason; Timeout input uint8; TRUE parameter; ComCANStop input; CANStopReason output Enum: enHeatStopReason

== stateflow chart Appl_HeatAdj_CtrlModel/LogicCtrl/LocalAdjustCtrl/LimitDeal/TimeoutFunction1/Timeout/TimeDiffTs/Chart ==
  (default) -> (junction 3)
  (junction 3) -> (junction 5)
  (junction 5) -> (junction 7) [order 1] : /* 入参比当前大 */
      | [lastTs > Ts]
  (junction 5) -> (junction 13) [order 2] : {OutTs = Ts - lastTs;}
  (junction 7) -> (junction 11) : {OutTs = 0xFFFFFFFF - lastTs + Ts +1;}
  (junction 11) -> (junction 13)
  (junction 13) -> (junction 17)
  data: lastTs input uint32; Ts input uint32; OutTs output uint32

== stateflow chart Appl_HeatAdj_CtrlModel/LogicCtrl/LocalAdjustCtrl/LimitDeal/TimeoutFunction2/Timeout ==
  state TimeCountStatus
    en,du:
    Level = enHeatLvlSts.EN_HEAT_LVL_OFF;
    TimeoutFlag = TRUE;
  state Default
    en,du:
    Level = InLevel;
    TimeoutFlag = FALSE;
  (default) -> Default
  Default -> TimeCountStatus : /*超时 */
      | [SwTimeout == TRUE]
  TimeCountStatus -> Default : /*无超时*/
      | [SwTimeout != TRUE]
      | /TimeoutFlag = FALSE;
  data: TimeoutPrm input uint8; TimeoutFlag output uint8; FALSE parameter; TRUE parameter; InLevel input Enum: enHeatLvlSts; MaxTime input uint32; Timer local uint32; Level output Enum: enHeatLvlSts; SwTimeout input

== stateflow chart Appl_HeatAdj_CtrlModel/LogicCtrl/LocalAdjustCtrl/LimitDeal/LevelLimitFunction1/LevelLimit ==
  state Default
    en:
    Level = enHeatLvlSts.EN_HEAT_LVL_OFF;
  state Run
    en:
    Level = OriginalLevel;
    CANStopReason = enHeatStopReason.EN_HEAT_STOP_R_NONE;
    du:
    Level = OriginalLevel;
  state ForbidStatus
    en:
    Level = enHeatLvlSts.EN_HEAT_LVL_OFF;
    CANStopReason = StopReason;
    //暂时屏蔽，查看是否需要一直保存禁能原因
    ex:
    StopReason = enHeatStopReason.EN_HEAT_STOP_R_NONE;
    (default) -> (junction 34)
    ForbidStatus -> (junction 34) [order 1]
    (junction 34) -> (junction 37) [order 1] : /*存在故障*/
        | [TRUE == Error]
    (junction 34) -> (junction 41) [order 2]
    (junction 37) -> (junction 39) : {StopReason = enHeatStopReason.EN_HEAT_STOP_R_FAULT;}
    (junction 39) -> (junction 41)
    (junction 41) -> (junction 44)
    (junction 44) -> (junction 46) [order 1] : /*互斥命令有效*/
        | [TRUE == OppositeCmd]
    (junction 44) -> (junction 50) [order 2]
    (junction 46) -> (junction 48) : {StopReason = enHeatStopReason.EN_HEAT_STOP_R_CMD;}
    (junction 48) -> (junction 50)
    (junction 50) -> (junction 62)
    (junction 62) -> (junction 60) [order 1] : /*恢复出厂*/
        | [TRUE == Heat_RecoverDefaultFlag]
    (junction 62) -> (junction 55) [order 2]
    (junction 60) -> (junction 58) : {StopReason = enHeatStopReason.EN_HEAT_STOP_R_FACTORY;}
    (junction 58) -> (junction 55)
    (junction 55) -> (junction 71)
    (junction 71) -> (junction 69) [order 1] : /*BM400掉线禁能*/
        | [TRUE == Heat_CanMessageLostFlag && enProjectType.EN_PROJECT_BM400 == CarType]
    (junction 71) -> (junction 67) [order 2]
    (junction 69) -> (junction 64) : {StopReason = enHeatStopReason.EN_HEAT_STOP_R_LOSS;}
    (junction 64) -> (junction 67)
    (junction 67) -> (junction 73)
  (default) -> Default
  ForbidStatus -> Default [order 1] : /*无用户请求，可准备下一轮禁能原因检测*/
      | [enHeatLvlSts.EN_HEAT_LVL_OFF == OriginalLevel]
  Default -> ForbidStatus : /*请求工作*/
      | [enHeatLvlSts.EN_HEAT_LVL_OFF != OriginalLevel]
  Run -> ForbidStatus [order 1] : /*存在故障*/
      | [TRUE == Error]
      | /StopReason = enHeatStopReason.EN_HEAT_STOP_R_FAULT;
  Run -> ForbidStatus [order 2] : /*互斥命令有效*/
      | [TRUE == OppositeCmd]
      | /StopReason = enHeatStopReason.EN_HEAT_STOP_R_CMD;
  Run -> ForbidStatus [order 3] : /*恢复出厂*/
      | [TRUE == Heat_RecoverDefaultFlag]
      | /StopReason = enHeatStopReason.EN_HEAT_STOP_R_FACTORY;
  Run -> ForbidStatus [order 4] : /*BM400掉线禁能*/
      | [TRUE == Heat_CanMessageLostFlag && enProjectType.EN_PROJECT_BM400 == CarType]
      | /StopReason = enHeatStopReason.EN_HEAT_STOP_R_LOSS;
  ForbidStatus -> Run [order 2] : /*无故障
      | && 互斥命令无效
      | && 无恢复出厂命令
      | && （BM400控制报文在线 || 非BM400车型）*/
      | [TRUE != Error ...
      | && TRUE != OppositeCmd ...
      | && TRUE != Heat_RecoverDefaultFlag ...
      | && ((FALSE == Heat_CanMessageLostFlag && enProjectType.EN_PROJECT_BM400 == CarType) ...
      | || (enProjectType.EN_PROJECT_BM400 != CarType))]
      | /StopReason = enHeatStopReason.EN_HEAT_STOP_R_NONE
  data: Level output Enum: enHeatLvlSts; StopReason output Enum: enHeatStopReason; OriginalLevel input Enum: enHeatLvlSts; Error input uint8; CarType input Enum: enProjectType; TRUE parameter; OppositeCmd input uint8; Heat_CanMessageLostFlag input uint8; Heat_RecoverDefaultFlag input uint8; FALSE parameter; CANStopReason output Enum: enHeatStopReason

== stateflow chart Appl_HeatAdj_CtrlModel/LogicCtrl/LocalAdjustCtrl/LimitDeal/LevelLimitFunction2/LevelLimit ==
  state Default
    en:
    Level = enHeatLvlSts.EN_HEAT_LVL_OFF;
  state Run
    en:
    Level = OriginalLevel;
    CANStopReason = enHeatStopReason.EN_HEAT_STOP_R_NONE;
    du:
    Level = OriginalLevel;
  state ForbidStatus
    en:
    Level = enHeatLvlSts.EN_HEAT_LVL_OFF;
    CANStopReason = StopReason;
    //暂时屏蔽，查看是否需要一直保存禁能原因
    ex:
    StopReason = enHeatStopReason.EN_HEAT_STOP_R_NONE;
    (default) -> (junction 34)
    ForbidStatus -> (junction 34) [order 1]
    (junction 34) -> (junction 37) [order 1] : /*存在故障*/
        | [TRUE == Error]
    (junction 34) -> (junction 41) [order 2]
    (junction 37) -> (junction 39) : {StopReason = enHeatStopReason.EN_HEAT_STOP_R_FAULT;}
    (junction 39) -> (junction 41)
    (junction 41) -> (junction 44)
    (junction 44) -> (junction 46) [order 1] : /*互斥命令有效*/
        | [TRUE == OppositeCmd]
    (junction 44) -> (junction 50) [order 2]
    (junction 46) -> (junction 48) : {StopReason = enHeatStopReason.EN_HEAT_STOP_R_CMD;}
    (junction 48) -> (junction 50)
    (junction 50) -> (junction 62)
    (junction 62) -> (junction 60) [order 1] : /*恢复出厂*/
        | [TRUE == Heat_RecoverDefaultFlag]
    (junction 62) -> (junction 55) [order 2]
    (junction 60) -> (junction 58) : {StopReason = enHeatStopReason.EN_HEAT_STOP_R_FACTORY;}
    (junction 58) -> (junction 55)
    (junction 55) -> (junction 71)
    (junction 71) -> (junction 69) [order 1] : /*BM400掉线禁能*/
        | [TRUE == Heat_CanMessageLostFlag && enProjectType.EN_PROJECT_BM400 == CarType]
    (junction 71) -> (junction 67) [order 2]
    (junction 69) -> (junction 64) : {StopReason = enHeatStopReason.EN_HEAT_STOP_R_LOSS;}
    (junction 64) -> (junction 67)
    (junction 67) -> (junction 73)
  (default) -> Default
  ForbidStatus -> Default [order 1] : /*无用户请求，可准备下一轮禁能原因检测*/
      | [enHeatLvlSts.EN_HEAT_LVL_OFF == OriginalLevel]
  Default -> ForbidStatus : /*请求工作*/
      | [enHeatLvlSts.EN_HEAT_LVL_OFF != OriginalLevel]
  Run -> ForbidStatus [order 1] : /*存在故障*/
      | [TRUE == Error]
      | /StopReason = enHeatStopReason.EN_HEAT_STOP_R_FAULT;
  Run -> ForbidStatus [order 2] : /*互斥命令有效*/
      | [TRUE == OppositeCmd]
      | /StopReason = enHeatStopReason.EN_HEAT_STOP_R_CMD;
  Run -> ForbidStatus [order 3] : /*恢复出厂*/
      | [TRUE == Heat_RecoverDefaultFlag]
      | /StopReason = enHeatStopReason.EN_HEAT_STOP_R_FACTORY;
  Run -> ForbidStatus [order 4] : /*BM400掉线禁能*/
      | [TRUE == Heat_CanMessageLostFlag && enProjectType.EN_PROJECT_BM400 == CarType]
      | /StopReason = enHeatStopReason.EN_HEAT_STOP_R_LOSS;
  ForbidStatus -> Run [order 2] : /*无故障
      | && 互斥命令无效
      | && 无恢复出厂命令
      | && （BM400控制报文在线 || 非BM400车型）*/
      | [TRUE != Error ...
      | && TRUE != OppositeCmd ...
      | && TRUE != Heat_RecoverDefaultFlag ...
      | && ((FALSE == Heat_CanMessageLostFlag && enProjectType.EN_PROJECT_BM400 == CarType) ...
      | || (enProjectType.EN_PROJECT_BM400 != CarType))]
      | /StopReason = enHeatStopReason.EN_HEAT_STOP_R_NONE
  data: Level output Enum: enHeatLvlSts; StopReason output Enum: enHeatStopReason; OriginalLevel input Enum: enHeatLvlSts; Error input uint8; CarType input Enum: enProjectType; TRUE parameter; OppositeCmd input uint8; Heat_CanMessageLostFlag input uint8; Heat_RecoverDefaultFlag input uint8; FALSE parameter; CANStopReason output Enum: enHeatStopReason

== stateflow chart Appl_HeatAdj_CtrlModel/LogicCtrl/LocalAdjustCtrl/LimitDeal/DiagnoseFunction1/Diagnose ==
  state Diagnose
    (default) -> (junction 6)
    Diagnose -> (junction 6)
    (junction 6) -> (junction 8) [order 1] : /* 无诊断指令 */
        | [0 == DiagCommand || DiagCommand > (enHeatLvlSts.EN_HEAT_LVL_3 + 1)]
    (junction 6) -> (junction 14) [order 2] : {Level = DiagCommand - 1;
        | Type = enHeatType.EN_HEAT_TYPE_DIAG;}
    (junction 8) -> (junction 10) : {Level = InLevel;
        | Type = CurrentType;}
    (junction 10) -> (junction 14)
    (junction 14) -> (junction 17)
  (default) -> Diagnose
  data: DiagCommand input uint8; InLevel input Enum: enHeatLvlSts; CurrentType input Enum: enHeatType; Level output Enum: enHeatLvlSts; Type output Enum: enHeatType

== stateflow chart Appl_HeatAdj_CtrlModel/LogicCtrl/LocalAdjustCtrl/LimitDeal/DiagnoseFunction2/Diagnose ==
  state Diagnose
    (default) -> (junction 6)
    Diagnose -> (junction 6)
    (junction 6) -> (junction 8) [order 1] : /* 无诊断指令 */
        | [0 == DiagCommand || DiagCommand > (enHeatLvlSts.EN_HEAT_LVL_3 + 1)]
    (junction 6) -> (junction 14) [order 2] : {Level = DiagCommand - 1;
        | Type = enHeatType.EN_HEAT_TYPE_DIAG;}
    (junction 8) -> (junction 10) : {Level = InLevel;
        | Type = CurrentType;}
    (junction 10) -> (junction 14)
    (junction 14) -> (junction 17)
  (default) -> Diagnose
  data: DiagCommand input uint8; InLevel input Enum: enHeatLvlSts; CurrentType input Enum: enHeatType; Level output Enum: enHeatLvlSts; Type output Enum: enHeatType

== stateflow chart Appl_HeatAdj_CtrlModel/LogicCtrl/LocalAdjustCtrl/OutputDeal/HeatOutFunction1/HeatOut ==
  state PwmCnt = PidGetPwm(CurrentTemp,SetTemp) [function]
  state Controll
    state None
      en:
      du:
      HeatOutGpio = OFF;
      HeatOutPwmCnt = 0;
      TimeCnt = 0;
    state AllOut
      en:
      du:
      HeatOutGpio = ON;
      HeatOutPwmCnt =100;
      TimeCnt = 0;
    state PwmOut
      en:
      HeatOutPwmCnt = PidGetPwm(CurrentTemp,SetTemp);
      (default) -> (junction 11)
      PwmOut -> (junction 11) [order 1]
      (junction 11) -> (junction 12) [order 1] : /* 100计数 */
          | [TimeCnt <= 100]
      (junction 11) -> (junction 15) [order 2] : /* 计算pid 算pwm */
          | {TimeCnt = 0;
          | HeatOutPwmCnt = PidGetPwm(CurrentTemp,SetTemp);}
      (junction 12) -> (junction 13) : {TimeCnt += 1;}
      (junction 13) -> (junction 14) [order 1] : [TimeCnt <= HeatOutPwmCnt]
      (junction 13) -> (junction 16) [order 2] : /* 引脚拉低 */
          | {HeatOutGpio = OFF;}
      (junction 14) -> (junction 17) : /* 引脚拉高 */
          | {HeatOutGpio = ON;}
      (junction 16) -> (junction 15)
      (junction 17) -> (junction 16)
      (junction 15) -> (junction 18)
    (default) -> None
    None -> AllOut [order 1] : /* 加热误差在3度 全开 */
        | [enHeatLvlSts.EN_HEAT_LVL_OFF < HeatLvl ...
        | && SetTemp > CurrentTemp ...
        | && (SetTemp - CurrentTemp) >= D_HEAT_HEAT_DEF]
    AllOut -> None [order 1] : /*全开 进 关 */
        | [SetTemp <= CurrentTemp ...
        | || enHeatLvlSts.EN_HEAT_LVL_OFF == HeatLvl]
    PwmOut -> AllOut [order 2] : /* 加热误差在3度 全开 */
        | [enHeatLvlSts.EN_HEAT_LVL_OFF < HeatLvl ...
        | && SetTemp > CurrentTemp ...
        | && (SetTemp - CurrentTemp) >= D_HEAT_HEAT_DEF]
    AllOut -> PwmOut [order 2] : /* 全开 进PID */
        | [enHeatLvlSts.EN_HEAT_LVL_OFF < HeatLvl ...
        | && SetTemp > CurrentTemp ...
        | && (SetTemp - CurrentTemp) < D_HEAT_HEAT_DEF]
    PwmOut -> None [order 1] : /* PID 进 关 */
        | [SetTemp <= CurrentTemp ...
        | || enHeatLvlSts.EN_HEAT_LVL_OFF == HeatLvl]
    None -> PwmOut [order 2] : /* 关 进 PID */
        | [enHeatLvlSts.EN_HEAT_LVL_OFF < HeatLvl ...
        | && SetTemp > CurrentTemp ...
        | && (SetTemp - CurrentTemp) < D_HEAT_HEAT_DEF]
  data: CurrentTemp function_input; PwmCnt function_output; SetTemp function_input; CurrentTemp input uint16; HeatLvl input Enum: enHeatLvlSts; SetTemp input uint16; HeatOutGpio output uint8; TimeCnt local uint8; OFF parameter; ON parameter; D_HEAT_HEAT_DEF parameter; HeatOutPwmCnt output uint8

== stateflow chart Appl_HeatAdj_CtrlModel/LogicCtrl/LocalAdjustCtrl/OutputDeal/HeatOutFunction1/HeatOut/PidGetPwm/Pid  ==
  (default) -> (junction 14)
  (junction 14) -> (junction 16) : /* 局部初始化 */
      | {Error = 0;
      | dError = 0;}
  (junction 16) -> (junction 20) : /* PID 计算 */
      | {Error = SetTemp - CurrentTemp;
      | SumError += Error;
      | dError = Error - LastError;
      | LastError = Error;
      | PwmCnt = (D_DRVHEAT_PID_P * Error)  + (D_DRVHEAT_PID_I *SumError) + (D_DRVHEAT_PID_D *  dError);}
  (junction 20) -> (junction 29) [order 1] : [PwmCnt > 100]
  (junction 20) -> (junction 27) [order 2]
  (junction 29) -> (junction 31) : {PwmCnt = 100;}
  (junction 31) -> (junction 27)
  (junction 27) -> (junction 34)
  data: dError local uint32; Error local uint32; CurrentTemp input uint16; SetTemp input uint16; PwmCnt output uint16; SumError local uint32; LastError local uint32; D_DRVHEAT_PID_P parameter; D_DRVHEAT_PID_I parameter; D_DRVHEAT_PID_D parameter
